simulink library "libc_filters_diff"  (R2013b)
settings: Solver=FixedStepDiscrete  StartTime=0.0  StopTime=Inf  FixedStep=0.004  RelTol=1e-3
PostLoadFcn:
  | , if any(exist('dsrtsu_mdlpostloadfcn', 'file') == [2, 3, 6]), try dsrtsu_mdlpostloadfcn('Execute', bdroot); catch fprintf('Error in PostLoadFcn (dsrtsu_mdlpostloadfcn) for model "%s":\n %s\n', bdroot, lasterr); end, end,
undefined symbols (not defined in the file or in its folder): accurate, CONST, dim, DiscIntNeverNeededParam, O
undefined symbols (not defined in the file): BHA
libraries: simulink x20, libc_filters_diff x8
settings Model: DSRTSU_INTERNAL_RTI_VER=440  DSRTSU_INTERNAL_RTI_TYPE=rti1005  DSRTSU_INTERNAL_RTIFPGA=30  Creator=Falkenhahn  LastModifiedBy=Falkenhahn

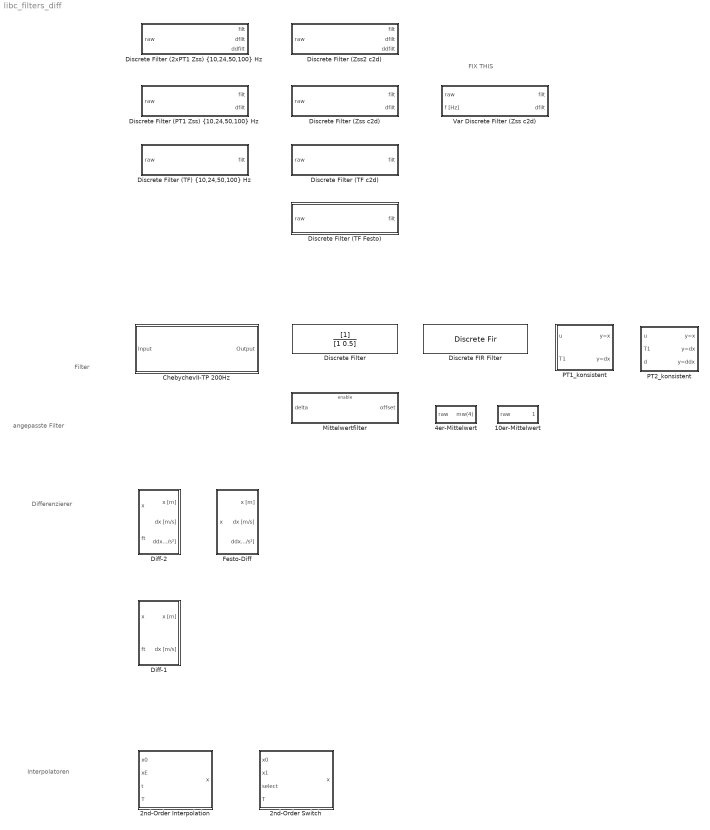
== system libc_filters_diff ==
  note: FIX THIS
  note: Filter
  note: Differenzierer
  note: angepasste Filter
  note: Interpolatoren
  10er-Mittelwert : Subsystem
      settings: AttributesFormatString=|
      | Mittelwert der
      | letzten 10 Werte
  2nd-Order Interpolation : Subsystem
  2nd-Order Switch : Subsystem
  4er-Mittelwert : Subsystem
      settings: AttributesFormatString=|
      | Mittelwert der
      | letzten 4 Werte
  ChebychevII-TP 200Hz : Subsystem  Tag=FilterWizardSubSystem  TreatAsAtomicUnit=on  SystemSampleTime=0.005
      settings: ErrorFcn=dspFilterRealizedInBasicElemsAlgLoopErrFcnCallback
      mask Display:
      | fprintf('Chebychev II-TP \n specified order: 4 \n F_Sample = 200 Hz \n F_Stopp = 25 Hz \n H_stopp^2<0.0001');
      | port_label('input', 1, 'vec-in');
      | port_label('output', 1, 'filt');
  Diff-1 : Subsystem  mask{fg=2.65}
      mask prompts: fg "Grenzfrequenz"
      mask help:
      | ft (feedthrough):
      | 0: phasengleichheit (maximal)
      | 1: phasenminimal
      settings: AttributesFormatString=f = %<fg>
  Diff-2 : Subsystem  mask{fg=2.65, D=1}
      mask prompts: fg "Grenzfrequenz fg"; D "Dämpfung D"
      mask help:
      | ft (feedthrough):
      | 0: phasengleichheit (maximal)
      | 1: phasenminimal
      |
      | D = 1 entspricht zwei PT1-Gliedern mit gleicher Zeitkonstante (kein Überschwingen)
      settings: AttributesFormatString=f = %<fg>\nD = %<D>
  Discrete FIR Filter : DiscreteFir
      settings: AttributesFormatString=sample time: %<SampleTime>
  Discrete Filter : DiscreteFilter
      settings: AttributesFormatString=sample time: %<SampleTime>
  "Discrete Filter (2xPT1 Zss) {10,24,50,100} Hz" : Subsystem  mask{rdnname2442_gf=10 Hz, rdnname2442_tA=CONST.tA}
      mask prompts: rdnname2442_gf "Grenzfrequenz"; rdnname2442_tA "Abstastzeit"
      mask init:
      | if rdnname2442_gf == 1 % first popup entry: 10 Hz
      |     rdnname2442_freq = 10;
      | elseif rdnname2442_gf == 2 % second popup entry: 24 Hz
      |     rdnname2442_freq = 24;
      | elseif rdnname2442_gf == 3 % third popup entry: 50 Hz
      |     rdnname2442_freq = 50;
      | else % rdnname2442_gf == 4 % third popup entry: 100 Hz
      |     rdnname2442_freq = 100;
      | end
      settings: AttributesFormatString=%<rdnname2442_gf>, tA: %<rdnname2442_tA>
      mask TypeOptions rdnname2442_gf: 10 Hz | 24 Hz | 50 Hz | 100 Hz
      mask Display: dpoly(1,[1/(2*pi*rdnname2442_freq) 1]);
  "Discrete Filter (PT1 Zss) {10,24,50,100} Hz" : Subsystem  mask{rdnname2442_gf=10 Hz, rdnname2442_tA=CONST.tA}
      mask prompts: rdnname2442_gf "Grenzfrequenz"; rdnname2442_tA "Abstastzeit"
      mask init: same as libc_filters_diff/Discrete Filter (2xPT1 Zss) {10,24,50,100} Hz
      settings: AttributesFormatString=%<rdnname2442_gf>, tA: %<rdnname2442_tA>
      mask TypeOptions rdnname2442_gf: 10 Hz | 24 Hz | 50 Hz | 100 Hz
      mask Display: dpoly(1,[1/(2*pi*rdnname2442_freq) 1])
  Discrete Filter (TF Festo) : Subsystem  mask{num_a=[1], den_a=[1/(2*pi*45), 1], Tsamp=CONST.tA, method='ramp', dar='z'}
      mask prompts: num_a "Numerator"; den_a "Denominator"; Tsamp "Abtastzeit, optional Abtastzeit für Diskret.  Ts  bzw.  [Ts,Ts_disk]"; method "Methode: Euler, Trapez, Heun, rK4, steP, step_U, Ramp, tr_100"; dar "Darstellung: z, z- = diskret, d = analoge ÜF des disk. Sys."
      mask init:
      | if length(Tsamp) == 0
      |     num_s = 0;
      |     num = 0;
      |     den_s = 1;
      |     den = 1;
      |     disp('ERROR: Abtastzeit nicht definiert. Ist CONST.tA definiert oder wurde die Abtastzeitvariable verändert?');
      | else
      |     Ts_int=Tsamp(1);
      |     if length(Tsamp)==1
      |         Ts=Tsamp(1); 
      |     else
      |         Ts=Tsamp(2);
      |     end
      |     if Ts == -1
      |         disp('ERROR: Abtastzeit für Diskretisierung = -1, Zweite Abtastzeit eingeben')
      |     end
      | 
      |     if exist('discret') == 2
      |         [a,b,c,d]=tf2ss(num_a,den_a); 
      |         [ad,bd,cd,dd,art]=discret(a,b,c,d,Ts,method,1e-9);
      |         [num,den]=ss2tf(ad,bd,cd,dd,1);
      |     else
      |         num_s = 0;
      |         num = 0;
      |         den_s = 1;
      |         den = 1;
      |         disp('ERROR: Festo tools initialisieren');
      |     end
      | 
      | 
      |     if dar(1) =='z'
      |         num_s=num; 
      |         den_s=den; 
      |     else
      |         num_s=num_a; 
      |         den_s=den_a; 
      |         if dar == 'd'
      |             dar = art
      |         end
      |     end
      | end
      settings: AttributesFormatString=sample time: %<Tsamp>
      mask Display:
      | if length(Tsamp) == 0
      |     disp('undefined sample time\n(e.g. CONST.tA)');
      | else
      |     if exist('discret') ~= 2
      |         disp('Festo tools not initialized');
      |     else
      |         dpoly(num_s,den_s,dar);
      |     end
      | end
  Discrete Filter (TF c2d) : Subsystem  mask(Diskretes Filter){rdnname2342_gf=45, rdnname2342_initial_cond=0, rdnname2342_tA=CONST.tA, rdnname2342_mode=noh (d=0), rdnname2342_showd=off}
      mask prompts: rdnname2342_gf "Grenzfrequenz [Hz]"; rdnname2342_initial_cond "Anfangsbedingungen"; rdnname2342_tA "Abtastzeit [s]"; rdnname2342_mode "Diskretisierung"; rdnname2342_showd "Diskrete Darstellung"
      mask init:
      | if rdnname2342_tA == 0
      |     error('invalid sample time');
      | end
      | if rdnname2342_gf == 0
      |     error('invalid cut-off frequency');
      | end
      | 
      | c_sys = tf(1,[1/(2*pi*rdnname2342_gf) 1]);
      | [rdnname2342_cnum,rdnname2342_cden] = tfdata(c_sys,'v');
      | 
      | rdnname2342_num = 1; % default value
      | rdnname2342_den = 1; % default value
      | if rdnname2342_mode == 3 % 'noh (d=0)'
      |     if exist('discret') == 2
      |         [a,b,c,d]=tf2ss(rdnname2342_cnum,rdnname2342_cden); 
      |         [ad,bd,cd,dd,art]=discret(a,b,c,d,rdnname2342_tA,'step_u',1e-9);
      |         [rdnname2342_num,rdnname2342_den]=ss2tf(ad,bd,cd,dd,1);
      |     else
      |         disp('ERROR: Festo tools initialisieren (fallback: foh (d=dt/2))'); 
      |         rdnname2342_mode = 2;
      |     end
      | end
      | if rdnname2342_mode == 2 % 'foh (d=dt/2)'
      |     d_sys = c2d(c_sys,rdnname2342_tA,'foh');
      |     [rdnname2342_num,rdnname2342_den] = tfdata(d_sys,'v');
      | end
      | if rdnname2342_mode == 1 % 'zoh (d=dt)'
      |     d_sys = c2d(c_sys,rdnname2342_tA);
      |     [rdnname2342_num,rdnname2342_den] = tfdata(d_sys,'v');
      | end
      settings: AttributesFormatString=%<rdnname2342_gf> Hz, IC: %<rdnname2342_initial_cond>, %<rdnname2342_mode>
      mask TypeOptions rdnname2342_mode: zoh (d=dt) | foh (d=dt/2) | noh (d=0)
      mask Display:
      | if rdnname2342_showd
      |     dpoly(rdnname2342_num,rdnname2342_den,'z')
      | else
      |     dpoly(rdnname2342_cnum,rdnname2342_cden);
      | end
  "Discrete Filter (TF) {10,24,50,100} Hz" : Subsystem  mask{rdnname2442_gf=10 Hz, rdnname2442_tA=CONST.tA, rdnname2442_IC=0}
      mask prompts: rdnname2442_gf "Grenzfrequenz"; rdnname2442_tA "Abstastzeit"; rdnname2442_IC "Anfangsbedingungen"
      mask init: same as libc_filters_diff/Discrete Filter (2xPT1 Zss) {10,24,50,100} Hz
      settings: AttributesFormatString=%<rdnname2442_gf>, IC: %<rdnname2442_IC>, tA: %<rdnname2442_tA>
      mask TypeOptions rdnname2442_gf: 10 Hz | 24 Hz | 50 Hz | 100 Hz
      mask Display: dpoly(1,[1/(2*pi*rdnname2442_freq) 1])
  Discrete Filter (Zss c2d) : Subsystem  mask(Diskretes Filter){rdnname2342_gf=45, rdnname2342_tA=CONST.tA, rdnname2342_mode=noh (d=0), rdnname2342_showd=on}
      mask prompts: rdnname2342_gf "Grenzfrequenz [Hz]"; rdnname2342_tA "Abtastzeit [s]"; rdnname2342_mode "Diskretisierung"; rdnname2342_showd "Diskrete Darstellung"
      mask init:
      | if rdnname2342_tA == 0
      |     error('invalid sample time');
      | end
      | if rdnname2342_gf == 0
      |     error('invalid cut-off frequency');
      | end
      | 
      | c_sys = tf(1,[1/(2*pi*rdnname2342_gf) 1]);
      | [rdnname2342_cnum,rdnname2342_cden] = tfdata(c_sys,'v');
      | 
      | rdnname2342_num = 1; % default value
      | rdnname2342_den = 1; % default value
      | if rdnname2342_mode == 3 % 'noh (d=0)'
      |     if exist('discret') == 2
      |         [a,b,c,d]=tf2ss(rdnname2342_cnum,rdnname2342_cden); 
      |         [ad,bd,cd,dd,art]=discret(a,b,c,d,rdnname2342_tA,'step_u',1e-9);
      |         [rdnname2342_num,rdnname2342_den]=ss2tf(ad,bd,cd,dd,1);
      |     else
      |         disp('ERROR: Festo tools initialisieren (fallback: foh (d=dt/2))'); 
      |         rdnname2342_mode = 2;
      |     end
      | end
      | if rdnname2342_mode == 2 % 'foh (d=dt/2)'
      |     d_sys = c2d(c_sys,rdnname2342_tA,'foh');
      |     [rdnname2342_num,rdnname2342_den] = tfdata(d_sys,'v');
      | end
      | if rdnname2342_mode == 1 % 'zoh (d=dt)'
      |     d_sys = c2d(c_sys,rdnname2342_tA);
      |     [rdnname2342_num,rdnname2342_den] = tfdata(d_sys,'v');
      | end
      | 
      | a = rdnname2342_den(2);
      | b = rdnname2342_den(1);
      | c = rdnname2342_num(2);
      | d = rdnname2342_num(1);
      settings: AttributesFormatString=%<rdnname2342_gf> Hz, %<rdnname2342_mode>
      mask TypeOptions rdnname2342_mode: zoh (d=dt) | foh (d=dt/2) | noh (d=0)
      mask Display:
      | if rdnname2342_showd
      |     dpoly(rdnname2342_num,rdnname2342_den,'z')
      | else
      |     dpoly(rdnname2342_cnum,rdnname2342_cden);
      | end
  Discrete Filter (Zss2 c2d) : Subsystem  mask(Diskretes Filter){rdnname2342_gf=45, rdnname2342_tA=CONST.tA, rdnname2342_mode=noh (d=0), rdnname2342_diffmode=O(2) [accurate], rdnname2342_showd=on}
      mask prompts: rdnname2342_gf "Grenzfrequenz [Hz]"; rdnname2342_tA "Abtastzeit [s]"; rdnname2342_mode "Diskretisierung"; rdnname2342_diffmode "Differenzierung"; rdnname2342_showd "Diskrete Darstellung"
      mask init: same as libc_filters_diff/Discrete Filter (Zss c2d)
      settings: AttributesFormatString=%<rdnname2342_gf> Hz, %<rdnname2342_mode>
      mask TypeOptions rdnname2342_mode: zoh (d=dt) | foh (d=dt/2) | noh (d=0)
      mask TypeOptions rdnname2342_diffmode: O(1) [low phase error] | O(2) [accurate]
      mask Display:
      | if rdnname2342_showd
      |     dpoly(rdnname2342_num,rdnname2342_den,'z');
      | else
      |     dpoly(rdnname2342_cnum,rdnname2342_cden);
      | end
  Festo-Diff : Subsystem
      settings: AttributesFormatString=mit PLC-Differenzierer
  Mittelwertfilter : Subsystem
      settings: AttributesFormatString=Eingangs-Mittelwertbildung wenn aktiviert,\nandernfalls wird Mittelwert gehalten & ausgegeben
  PT1_konsistent : Subsystem
  PT2_konsistent : Subsystem
  Var Discrete Filter (Zss c2d) : Subsystem  mask(Diskretes Filter){rdnname2342_tA=CONST.tA, rdnname2342_mode=noh (d=0)}
      mask prompts: rdnname2342_tA "Abtastzeit [s]"; rdnname2342_mode "Diskretisierung"
      mask init:
      | if rdnname2342_tA == 0
      |     error('invalid sample time');
      | end
      settings: AttributesFormatString=|
      | %<rdnname2342_mode>
      | CURRENTLY NOT USABLE FOR CODE GENERATION
      | BODE / C2D / TF ...
      mask TypeOptions rdnname2342_mode: zoh (d=dt) | foh (d=dt/2) | noh (d=0)
      mask Display: fprintf('!!!  FIX  ME !!!');

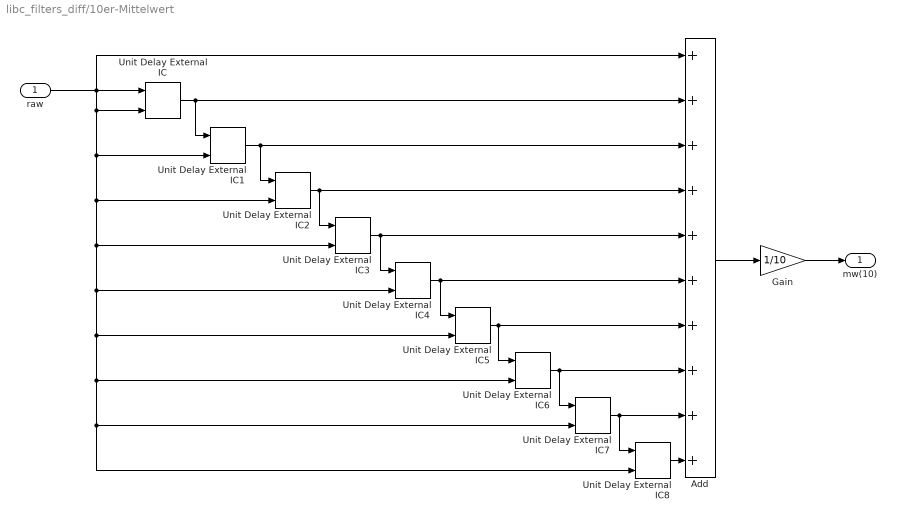
== system libc_filters_diff/10er-Mittelwert ==
  raw : Inport
  Add : Sum  Inputs=10
  Gain : Gain  Gain=1/10
  Unit Delay External IC{,1..8} (9 alike) : simulink/Additional Math & Discrete/Additional Discrete/Unit Delay External IC  tsamp=-1
  mw(10) : Outport  InitialOutput=zeros(1,dim)
  wires:
  Gain/1 -> mw(10)/1
  Add/1 -> Gain/1
  Unit Delay External IC2/1 -> Unit Delay External IC3/1, Add/4
  Unit Delay External IC1/1 -> Unit Delay External IC2/1, Add/3
  Unit Delay External IC/1 -> Add/2, Unit Delay External IC1/1
  raw/1 -> Unit Delay External IC/1, Add/1, Unit Delay External IC/2, Unit Delay External IC3/2, Unit Delay External IC4/2, Unit Delay External IC5/2, Unit Delay External IC6/2, Unit Delay External IC7/2, Unit Delay External IC8/2, Unit Delay External IC2/2, Unit Delay External IC1/2
  Unit Delay External IC8/1 -> Add/10
  Unit Delay External IC7/1 -> Add/9, Unit Delay External IC8/1
  Unit Delay External IC6/1 -> Add/8, Unit Delay External IC7/1
  Unit Delay External IC5/1 -> Unit Delay External IC6/1, Add/7
  Unit Delay External IC4/1 -> Unit Delay External IC5/1, Add/6
  Unit Delay External IC3/1 -> Add/5, Unit Delay External IC4/1

== system libc_filters_diff/2nd-Order Interpolation ==
  x0 : Inport
  xE : Inport  Port=2
  t : Inport  Port=3
  T : Inport  Port=4
  2nd-Order Interpolation : MATLAB Function  TreatAsAtomicUnit=on
  x : Outport
  wires:
  t/1 -> 2nd-Order Interpolation/3(t)
  2nd-Order Interpolation/1(x) -> x/1
  x0/1 -> 2nd-Order Interpolation/1(x0)
  xE/1 -> 2nd-Order Interpolation/2(xE)
  T/1 -> 2nd-Order Interpolation/4(T)

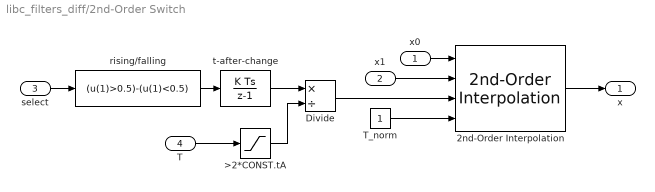
== system libc_filters_diff/2nd-Order Switch ==
  x0 : Inport
  x1 : Inport  Port=2
  select : Inport  Port=3
  T : Inport  Port=4
  2nd-Order Interpolation : libc_filters_diff/2nd-Order Interpolation
  >2*CONST.tA : Saturate  UpperLimit=inf  LowerLimit=2*CONST.tA
  Divide : Product  Inputs=*/
  T_norm : Constant
  rising/falling : Fcn  Expr=(u(1)>0.5)-(u(1)<0.5)
  t-after-change : DiscreteIntegrator  SampleTime=-1  LimitOutput=on  UpperSaturationLimit=1  LowerSaturationLimit=0  ICPrevOutput=DiscIntNeverNeededParam  ICPrevScaledInput=DiscIntNeverNeededParam
  x : Outport
  wires:
  2nd-Order Interpolation/1 -> x/1
  x0/1 -> 2nd-Order Interpolation/1
  x1/1 -> 2nd-Order Interpolation/2
  select/1 -> rising/falling/1
  Divide/1 -> 2nd-Order Interpolation/3
  rising/falling/1 -> t-after-change/1
  T_norm/1 -> 2nd-Order Interpolation/4
  >2*CONST.tA/1 -> Divide/2
  T/1 -> >2*CONST.tA/1
  t-after-change/1 -> Divide/1

== system libc_filters_diff/4er-Mittelwert ==
  raw : Inport
  Add : Sum  Inputs=++++
  Gain : Gain  Gain=1/4
  Unit Delay External IC : simulink/Additional Math & Discrete/Additional Discrete/Unit Delay External IC  tsamp=-1
  Unit Delay External IC1 : simulink/Additional Math & Discrete/Additional Discrete/Unit Delay External IC  tsamp=-1
  Unit Delay External IC2 : simulink/Additional Math & Discrete/Additional Discrete/Unit Delay External IC  tsamp=-1
  mw(4) : Outport  InitialOutput=zeros(1,dim)
  wires:
  raw/1 -> Unit Delay External IC1/2, Unit Delay External IC2/2, Unit Delay External IC/2, Add/1, Unit Delay External IC/1
  Unit Delay External IC/1 -> Unit Delay External IC1/1, Add/2
  Unit Delay External IC1/1 -> Add/3, Unit Delay External IC2/1
  Unit Delay External IC2/1 -> Add/4
  Add/1 -> Gain/1
  Gain/1 -> mw(4)/1

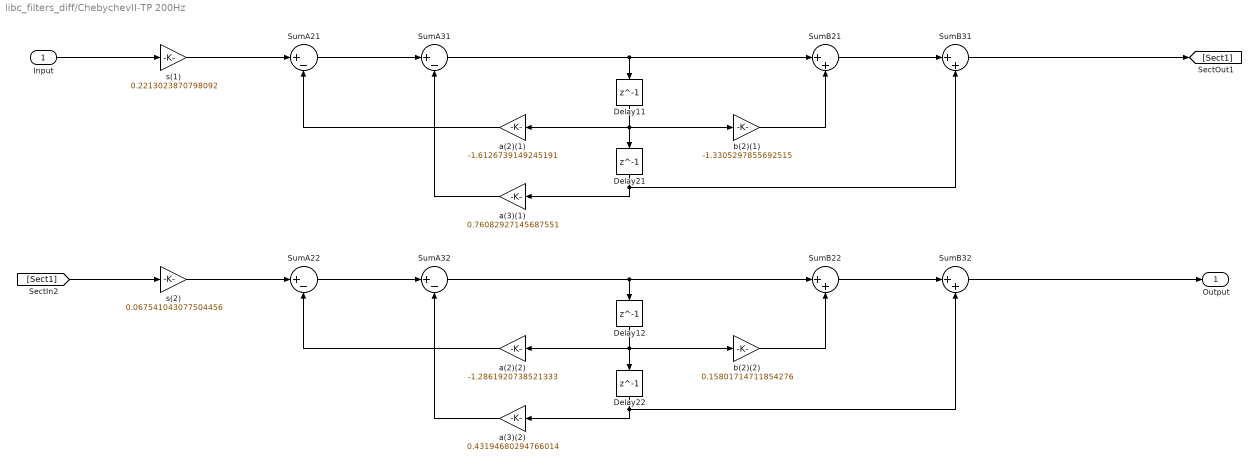
== system libc_filters_diff/ChebychevII-TP 200Hz ==
  Input : Inport
  Delay{11..12,21..22} (4 alike) : Delay  DelayLength=1  InitialCondition=0  InputProcessing=Inherited
  SumA{21..22,31..32} (4 alike) : Sum  Inputs=|+-  RndMeth=Nearest  SaturateOnIntegerOverflow=on  OutDataTypeStr=Inherit: Same as first input
  SumB{21..22,31..32} (4 alike) : Sum  Inputs=|++  RndMeth=Nearest  SaturateOnIntegerOverflow=on  OutDataTypeStr=Inherit: Same as first input
  a(2)(1) : Gain  Gain=-1.6126739149245191  ParamDataTypeStr=float('double')  RndMeth=Nearest  SaturateOnIntegerOverflow=on  OutDataTypeStr=Inherit: Same as input
  a(2)(2) : Gain  Gain=-1.2861920738521333  ParamDataTypeStr=float('double')  RndMeth=Nearest  SaturateOnIntegerOverflow=on  OutDataTypeStr=Inherit: Same as input
  a(3)(1) : Gain  Gain=0.76082927145687551  ParamDataTypeStr=float('double')  RndMeth=Nearest  SaturateOnIntegerOverflow=on  OutDataTypeStr=Inherit: Same as input
  a(3)(2) : Gain  Gain=0.43194680294766014  ParamDataTypeStr=float('double')  RndMeth=Nearest  SaturateOnIntegerOverflow=on  OutDataTypeStr=Inherit: Same as input
  b(2)(1) : Gain  Gain=-1.3305297855692515  ParamDataTypeStr=float('double')  RndMeth=Nearest  SaturateOnIntegerOverflow=on  OutDataTypeStr=Inherit: Same as input
  b(2)(2) : Gain  Gain=0.15801714711854276  ParamDataTypeStr=float('double')  RndMeth=Nearest  SaturateOnIntegerOverflow=on  OutDataTypeStr=Inherit: Same as input
  s(1) : Gain  Gain=0.2213023870798092  ParamDataTypeStr=float('double')  RndMeth=Nearest  SaturateOnIntegerOverflow=on  OutDataTypeStr=Inherit: Same as input
  s(2) : Gain  Gain=0.067541043077504456  ParamDataTypeStr=float('double')  RndMeth=Nearest  SaturateOnIntegerOverflow=on  OutDataTypeStr=Inherit: Same as input
  Output : Outport
  wires:
  Delay22/1 -> SumB32/2, a(3)(2)/1
  a(3)(2)/1 -> SumA32/2
  b(2)(2)/1 -> SumB22/2
  Delay12/1 -> Delay22/1, b(2)(2)/1, a(2)(2)/1
  a(2)(2)/1 -> SumA22/2
  SumB32/1 -> Output/1
  SumB22/1 -> SumB32/1
  SumA32/1 -> Delay12/1, SumB22/1
  SumA22/1 -> SumA32/1
  s(2)/1 -> SumA22/1
  [Sect1] -> s(2)/1
  Delay21/1 -> SumB31/2, a(3)(1)/1
  a(3)(1)/1 -> SumA31/2
  b(2)(1)/1 -> SumB21/2
  Delay11/1 -> Delay21/1, b(2)(1)/1, a(2)(1)/1
  a(2)(1)/1 -> SumA21/2
  SumB31/1 -> [Sect1]
  SumB21/1 -> SumB31/1
  SumA31/1 -> Delay11/1, SumB21/1
  SumA21/1 -> SumA31/1
  s(1)/1 -> SumA21/1
  Input/1 -> s(1)/1

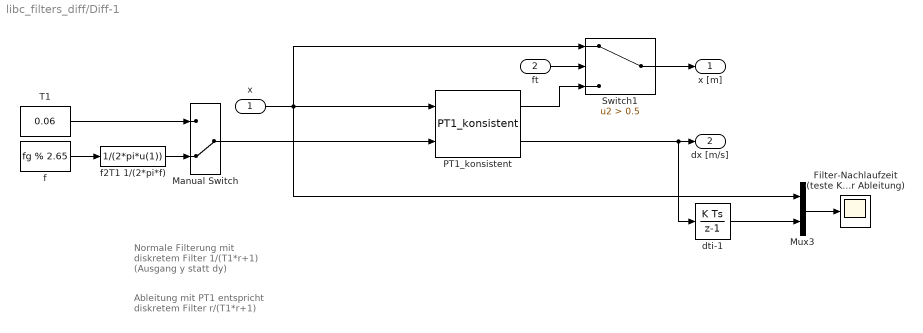
== system libc_filters_diff/Diff-1 ==
  note: Normale Filterung mit
      | diskretem Filter 1/(T1*r+1)
      | (Ausgang y statt dy)
  note: Ableitung mit PT1 entspricht
      | diskretem Filter r/(T1*r+1)
  x : Inport
  ft : Inport  Port=2
  Filter-Nachlaufzeit (teste Konsistenz der Ableitung) : Scope
      settings: TimeRange=10  YMin=0.22  YMax=0.2625  SaveName=ScopeData6
  Manual Switch : ManualSwitch  CurrentSetting=0
  Mux3 : Mux  Inputs=2
  PT1_konsistent : libc_filters_diff/PT1_konsistent
  Switch1 : Switch  Criteria=u2 > Threshold  Threshold=0.5
  T1 : Constant  Value=0.06
  dti-1 : DiscreteIntegrator  SampleTime=-1  ICPrevOutput=DiscIntNeverNeededParam  ICPrevScaledInput=DiscIntNeverNeededParam
  f : Constant  Value=fg % 2.65
  f2T1 1/(2*pi*f) : Fcn  Expr=1/(2*pi*u(1))
  x [m] : Outport
  dx [m/s] : Outport  Port=2
  wires:
  PT1_konsistent/2 -> dti-1/1, dx [m/s]/1
  Switch1/1 -> x [m]/1
  ft/1 -> Switch1/2
  f/1 -> f2T1 1/(2*pi*f)/1
  f2T1 1/(2*pi*f)/1 -> Manual Switch/2
  T1/1 -> Manual Switch/1
  x/1 -> Mux3/1, Switch1/1, PT1_konsistent/1
  dti-1/1 -> Mux3/2
  Mux3/1 -> Filter-Nachlaufzeit (teste Konsistenz der Ableitung)/1
  PT1_konsistent/1 -> Switch1/3
  Manual Switch/1 -> PT1_konsistent/2

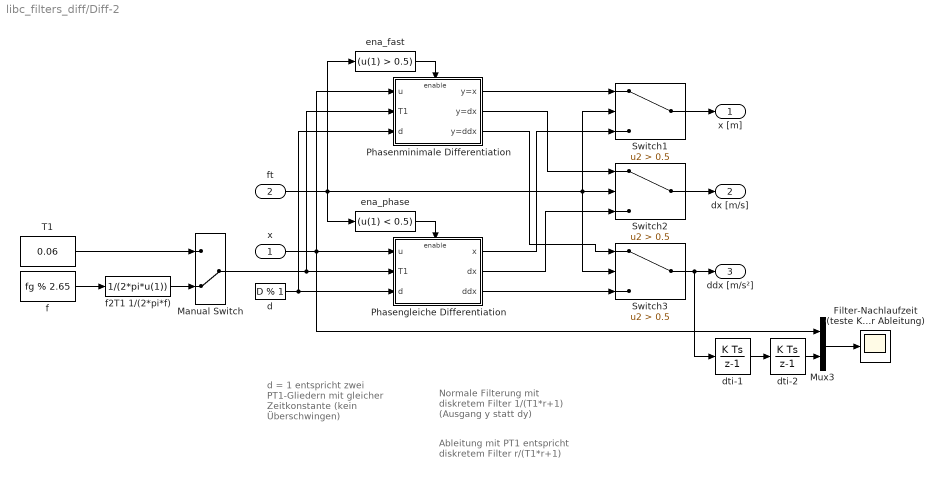
== system libc_filters_diff/Diff-2 ==
  note: Ableitung mit PT1 entspricht
      | diskretem Filter r/(T1*r+1)
  note: Normale Filterung mit
      | diskretem Filter 1/(T1*r+1)
      | (Ausgang y statt dy)
  note: d = 1
      | entspricht zwei PT1-Gliedern mit
      | gleicher Zeitkonstante
      | (kein Überschwingen)
  x : Inport
  ft : Inport  Port=2
  Filter-Nachlaufzeit (teste Konsistenz der Ableitung) : Scope
      settings: TimeRange=10  YMin=0.22  YMax=0.2625  SaveName=ScopeData6
  Manual Switch : ManualSwitch  CurrentSetting=0
  Mux3 : Mux  Inputs=2
  Phasengleiche Differentiation : Subsystem
  Phasenminimale Differentiation : Subsystem
  Switch1 : Switch  Criteria=u2 > Threshold  Threshold=0.5
  Switch2 : Switch  Criteria=u2 > Threshold  Threshold=0.5
  Switch3 : Switch  Criteria=u2 > Threshold  Threshold=0.5
  T1 : Constant  Value=0.06
  d : Constant  Value=D % 1
  dti-1 : DiscreteIntegrator  SampleTime=-1  ICPrevOutput=DiscIntNeverNeededParam  ICPrevScaledInput=DiscIntNeverNeededParam
  dti-2 : DiscreteIntegrator  SampleTime=-1  ICPrevOutput=DiscIntNeverNeededParam  ICPrevScaledInput=DiscIntNeverNeededParam
  ena_fast : Fcn  Expr=(u(1) > 0.5)
  ena_phase : Fcn  Expr=(u(1) < 0.5)
  f : Constant  Value=fg % 2.65
  f2T1 1/(2*pi*f) : Fcn  Expr=1/(2*pi*u(1))
  x [m] : Outport
  dx [m/s] : Outport  Port=2
  ddx [m/s²] : Outport  Port=3
  wires:
  Mux3/1 -> Filter-Nachlaufzeit (teste Konsistenz der Ableitung)/1
  dti-2/1 -> Mux3/2
  dti-1/1 -> dti-2/1
  x/1 -> Mux3/1, Phasenminimale Differentiation/1(u), Phasengleiche Differentiation/1(u)
  T1/1 -> Manual Switch/1
  f2T1 1/(2*pi*f)/1 -> Manual Switch/2
  f/1 -> f2T1 1/(2*pi*f)/1
  Manual Switch/1 -> Phasenminimale Differentiation/2(T1), Phasengleiche Differentiation/2(T1)
  d/1 -> Phasenminimale Differentiation/3(d), Phasengleiche Differentiation/3(d)
  Phasenminimale Differentiation/1(y=x) -> Switch1/1
  Phasengleiche Differentiation/1(x) -> Switch1/3
  Phasengleiche Differentiation/3(ddx) -> Switch3/3
  Phasengleiche Differentiation/2(dx) -> Switch2/3
  Phasenminimale Differentiation/2(y=dx) -> Switch2/1
  Phasenminimale Differentiation/3(y=ddx) -> Switch3/1
  ena_fast/1 -> Phasenminimale Differentiation/Enable
  ena_phase/1 -> Phasengleiche Differentiation/Enable
  ft/1 -> ena_fast/1, Switch3/2, Switch1/2, Switch2/2, ena_phase/1
  Switch1/1 -> x [m]/1
  Switch2/1 -> dx [m/s]/1
  Switch3/1 -> dti-1/1, ddx [m/s²]/1

== system libc_filters_diff/Discrete Filter (2xPT1 Zss) {10,24,50,100} Hz ==
  note: zum Filtern am besten geeignet
      | (da kein Phasenverlust): noh (d=0)
  raw : Inport
  Discrete Filter (Zss2 c2d) : libc_filters_diff/Discrete Filter (Zss2 c2d)  rdnname2342_gf=rdnname2442_freq  rdnname2342_tA=rdnname2442_tA  rdnname2342_mode=noh (d=0)  rdnname2342_diffmode=O(2) [accurate]  rdnname2342_showd=on
      settings: AttributesFormatString=%<rdnname2342_gf> Hz, %<rdnname2342_mode>
  filt : Outport
  dfilt : Outport  Port=2
  ddfilt : Outport  Port=3
  wires:
  Discrete Filter (Zss2 c2d)/2 -> dfilt/1
  raw/1 -> Discrete Filter (Zss2 c2d)/1
  Discrete Filter (Zss2 c2d)/1 -> filt/1
  Discrete Filter (Zss2 c2d)/3 -> ddfilt/1

== system libc_filters_diff/Discrete Filter (PT1 Zss) {10,24,50,100} Hz ==
  note: zum Filtern am besten geeignet
      | (da kein Phasenverlust): noh (d=0)
  raw : Inport
  Discrete Filter (Zss c2d) : libc_filters_diff/Discrete Filter (Zss c2d)  rdnname2342_gf=rdnname2442_freq  rdnname2342_tA=rdnname2442_tA  rdnname2342_mode=noh (d=0)  rdnname2342_showd=on
      settings: AttributesFormatString=%<rdnname2342_gf> Hz, %<rdnname2342_mode>
  filt : Outport
  dfilt : Outport  Port=2
  wires:
  Discrete Filter (Zss c2d)/1 -> filt/1
  raw/1 -> Discrete Filter (Zss c2d)/1
  Discrete Filter (Zss c2d)/2 -> dfilt/1

== system libc_filters_diff/Discrete Filter (TF Festo) ==
  raw : Inport
  Discrete Transfer Fcn : DiscreteTransferFcn  Numerator=num  Denominator=den  SampleTime=Ts_int
  filt : Outport
  wires:
  raw/1 -> Discrete Transfer Fcn/1
  Discrete Transfer Fcn/1 -> filt/1

== system libc_filters_diff/Discrete Filter (TF c2d) ==
  raw : Inport
  Diskretes Filter : DiscreteTransferFcn  Numerator=rdnname2342_num  Denominator=rdnname2342_den  InitialStates=rdnname2342_initial_cond  ExternalReset=Rising  SampleTime=rdnname2342_tA
      settings: InputPortMap=u0,r7
  reset : Constant  Value=0
  filt : Outport
  wires:
  reset/1 -> Diskretes Filter/2
  raw/1 -> Diskretes Filter/1
  Diskretes Filter/1 -> filt/1

== system libc_filters_diff/Discrete Filter (TF) {10,24,50,100} Hz ==
  note: zum Filtern am besten geeignet
      | (da kein Phasenverlust): noh (d=0)
  raw : Inport
  Discrete Filter (TF c2d) : libc_filters_diff/Discrete Filter (TF c2d)  rdnname2342_gf=rdnname2442_freq  rdnname2342_initial_cond=rdnname2442_IC  rdnname2342_tA=rdnname2442_tA  rdnname2342_mode=noh (d=0)  rdnname2342_showd=on
      settings: AttributesFormatString=%<rdnname2342_gf> Hz, IC: %<rdnname2342_initial_cond>, %<rdnname2342_mode>
  filt : Outport
  wires:
  raw/1 -> Discrete Filter (TF c2d)/1
  Discrete Filter (TF c2d)/1 -> filt/1

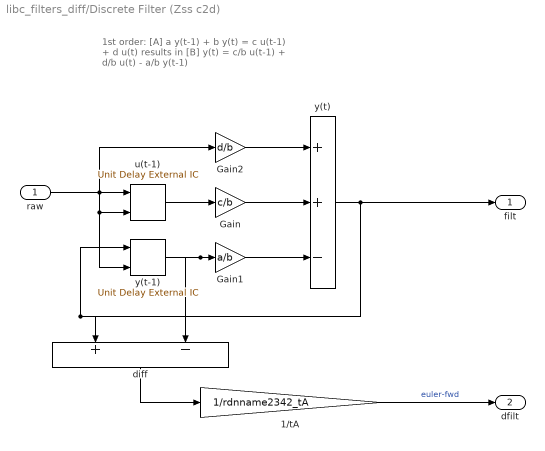
== system libc_filters_diff/Discrete Filter (Zss c2d) ==
  note: 1st order:
      | [A]  a y(t-1) + b y(t) = c u(t-1) + d u(t)
      | results in
      | [B]  y(t) = c/b u(t-1) + d/b u(t) - a/b y(t-1)
  raw : Inport
  1/tA : Gain  Gain=1/rdnname2342_tA
  Gain : Gain  Gain=c/b
  Gain1 : Gain  Gain=a/b
  Gain2 : Gain  Gain=d/b
  diff : Sum  Inputs=+|-
  u(t-1) : simulink/Additional Math & Discrete/Additional Discrete/Unit Delay External IC  tsamp=rdnname2342_tA
  y(t) : Sum  Inputs=++-
  y(t-1) : simulink/Additional Math & Discrete/Additional Discrete/Unit Delay External IC  tsamp=rdnname2342_tA
  filt : Outport
  dfilt : Outport  Port=2
  wires:
  1/tA/1 -> dfilt/1  "euler-fwd"
  diff/1 -> 1/tA/1
  raw/1 -> u(t-1)/1, u(t-1)/2, y(t-1)/2, Gain2/1
  y(t)/1 -> diff/1, y(t-1)/1, filt/1
  Gain1/1 -> y(t)/3
  Gain/1 -> y(t)/2
  Gain2/1 -> y(t)/1
  y(t-1)/1 -> diff/2, Gain1/1
  u(t-1)/1 -> Gain/1

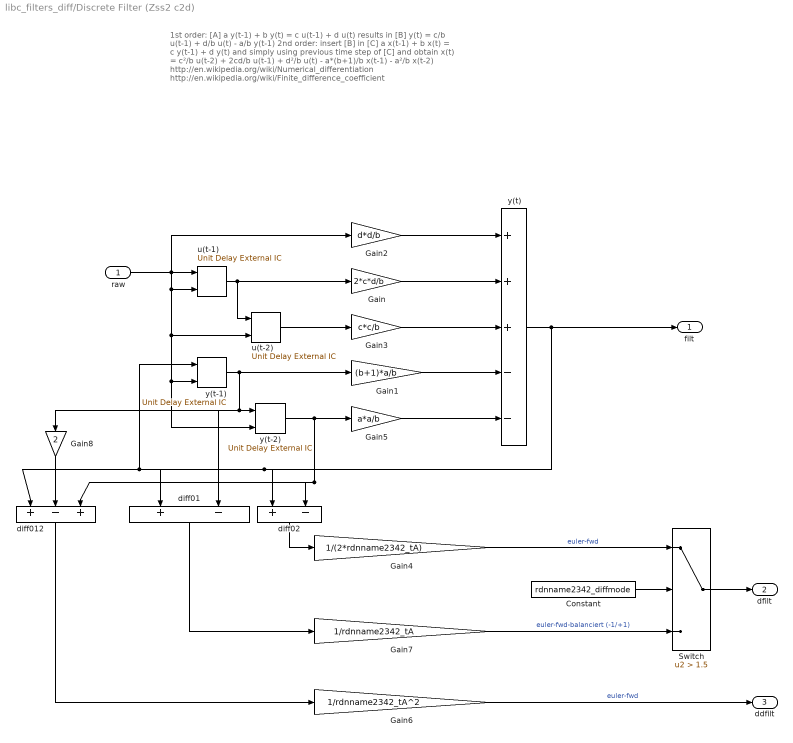
== system libc_filters_diff/Discrete Filter (Zss2 c2d) ==
  note: 1st order:
      | [A]  a y(t-1) + b y(t) = c u(t-1) + d u(t)
      | results in
      | [B]  y(t) = c/b u(t-1) + d/b u(t) - a/b y(t-1)
      |
      | 2nd order:  insert [B] in
      | [C]  a x(t-1) + b x(t) = c y(t-1) + d y(t)
      | and simply using previous time step of [C] and obtain
      | x(t) = c²/b u(t-2) + 2cd/b u(t-1) + d²/b u(t) - a*(b+1)/b x(t-1) - a²/b x(t-2)
      |
      | http://en.wikipedia.org/wiki/Numerical_differentiation
      | http://en.wikipedia.org/wiki/Finite_difference_coefficient
  raw : Inport
  Constant : Constant  Value=rdnname2342_diffmode
  Gain : Gain  Gain=2*c*d/b
  Gain1 : Gain  Gain=(b+1)*a/b
  Gain2 : Gain  Gain=d*d/b
  Gain3 : Gain  Gain=c*c/b
  Gain4 : Gain  Gain=1/(2*rdnname2342_tA)
  Gain5 : Gain  Gain=a*a/b
  Gain6 : Gain  Gain=1/rdnname2342_tA^2
  Gain7 : Gain  Gain=1/rdnname2342_tA
  Gain8 : Gain  Gain=2
  Switch : Switch  Criteria=u2 > Threshold  Threshold=1.5
  diff01 : Sum  Inputs=+|||-
  diff012 : Sum  Inputs=+|-|+
  diff02 : Sum  Inputs=+|||-
  u(t-1) : simulink/Additional Math & Discrete/Additional Discrete/Unit Delay External IC  tsamp=rdnname2342_tA
  u(t-2) : simulink/Additional Math & Discrete/Additional Discrete/Unit Delay External IC  tsamp=rdnname2342_tA
  y(t) : Sum  Inputs=+++--
  y(t-1) : simulink/Additional Math & Discrete/Additional Discrete/Unit Delay External IC  tsamp=rdnname2342_tA
  y(t-2) : simulink/Additional Math & Discrete/Additional Discrete/Unit Delay External IC  tsamp=rdnname2342_tA
  filt : Outport
  dfilt : Outport  Port=2
  ddfilt : Outport  Port=3
  wires:
  u(t-1)/1 -> u(t-2)/1, Gain/1
  y(t-1)/1 -> Gain1/1, Gain8/1, diff01/2, y(t-2)/1
  y(t)/1 -> y(t-1)/1, diff01/1, diff012/1, diff02/1, filt/1
  raw/1 -> Gain2/1, y(t-1)/2, y(t-2)/2, u(t-2)/2, u(t-1)/2, u(t-1)/1
  diff02/1 -> Gain4/1
  Gain4/1 -> Switch/1  "euler-fwd"
  u(t-2)/1 -> Gain3/1
  y(t-2)/1 -> Gain5/1, diff012/3, diff02/2
  Gain1/1 -> y(t)/4
  Gain3/1 -> y(t)/3
  Gain/1 -> y(t)/2
  Gain2/1 -> y(t)/1
  Gain5/1 -> y(t)/5
  Gain6/1 -> ddfilt/1  "euler-fwd"
  diff01/1 -> Gain7/1
  Gain7/1 -> Switch/3  "euler-fwd-balanciert (-1/+1)"
  Switch/1 -> dfilt/1
  Gain8/1 -> diff012/2
  diff012/1 -> Gain6/1
  Constant/1 -> Switch/2

== system libc_filters_diff/Festo-Diff ==
  x : Inport
  For Each Subsystem : Subsystem  TreatAsAtomicUnit=on
  Permute Dimensions : PermuteDimensions
  Permute Dimensions1 : PermuteDimensions
  Selector : Selector  NumberOfDimensions=2  InputPortWidth=3  IndexOptions=Index vector (dialog),Select all  Indices=[1],1  OutputSizes=1,1
  Selector1 : Selector  NumberOfDimensions=2  InputPortWidth=3  IndexOptions=Index vector (dialog),Select all  Indices=[2],1  OutputSizes=1,1
  x [m] : Outport
  dx [m/s] : Outport  Port=2
  ddx [m/s²] : Outport  Port=3
  wires:
  Permute Dimensions1/1 -> dx [m/s]/1
  Permute Dimensions/1 -> ddx [m/s²]/1
  Selector1/1 -> Permute Dimensions/1
  For Each Subsystem/1("[x dx ddx]") -> Selector/1, Selector1/1
  x/1 -> For Each Subsystem/1(x), x [m]/1
  Selector/1 -> Permute Dimensions1/1

== system libc_filters_diff/Mittelwertfilter ==
  delta : Inport
  Enable : EnablePort  StatesWhenEnabling=reset
  Add1 : Sum  Inputs=+++
  Add2 : Sum
  Constant : Constant
  Divide : Product  Inputs=*/
  Unit Delay : UnitDelay  SampleTime=-1
  Unit Delay2 : UnitDelay  SampleTime=-1
  size : Gain  Gain=0
  offset : Outport  InitialOutput=0
  wires:
  size/1 -> Add1/1
  Constant/1 -> Add1/2
  Add1/1 -> Divide/2, Unit Delay2/1
  Unit Delay2/1 -> Add1/3
  Add2/1 -> Unit Delay/1, Divide/1
  Unit Delay/1 -> Add2/2
  delta/1 -> Add2/1, size/1
  Divide/1 -> offset/1

== system libc_filters_diff/PT1_konsistent ==
  u : Inport
  T1 : Inport  Port=2
  Add2 : Sum  Inputs=+-
  Product : Product  Inputs=*/  RndMeth=Zero
  dti2 : DiscreteIntegrator  InitialConditionSource=external  SampleTime=-1  ICPrevOutput=DiscIntNeverNeededParam  ICPrevScaledInput=DiscIntNeverNeededParam
  y=x : Outport
  y=dx : Outport  Port=2
  wires:
  u/1 -> Add2/1, dti2/2
  dti2/1 -> y=x/1, Add2/2
  Add2/1 -> Product/1
  T1/1 -> Product/2
  Product/1 -> dti2/1, y=dx/1

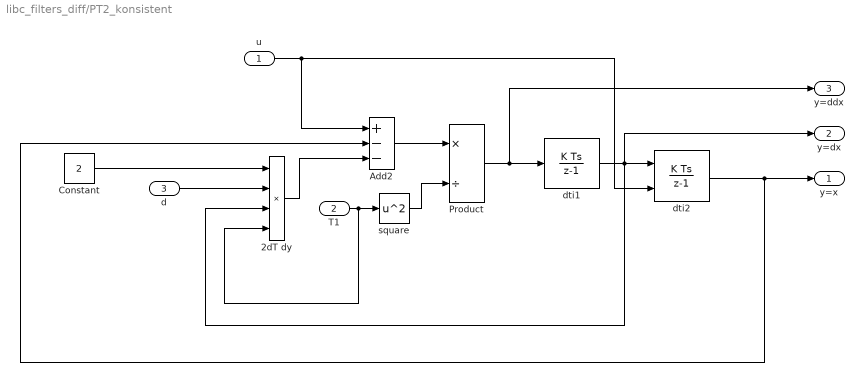
== system libc_filters_diff/PT2_konsistent ==
  u : Inport
  T1 : Inport  Port=2
  d : Inport  Port=3
  2dT dy : Product  Inputs=****  RndMeth=Zero
  Add2 : Sum  Inputs=+--
  Constant : Constant  Value=2
  Product : Product  Inputs=*/  RndMeth=Zero
  dti1 : DiscreteIntegrator  SampleTime=-1  ICPrevOutput=DiscIntNeverNeededParam  ICPrevScaledInput=DiscIntNeverNeededParam
  dti2 : DiscreteIntegrator  InitialConditionSource=external  InitialCondition=0.174  SampleTime=-1  ICPrevOutput=DiscIntNeverNeededParam  ICPrevScaledInput=DiscIntNeverNeededParam
  square : Math  Operator=square  SaturateOnIntegerOverflow=on
  y=x : Outport
  y=dx : Outport  Port=2
  y=ddx : Outport  Port=3
  wires:
  d/1 -> 2dT dy/2
  Constant/1 -> 2dT dy/1
  2dT dy/1 -> Add2/3
  square/1 -> Product/2
  dti1/1 -> dti2/1, y=dx/1, 2dT dy/3
  T1/1 -> 2dT dy/4, square/1
  Add2/1 -> Product/1
  Product/1 -> dti1/1, y=ddx/1
  dti2/1 -> Add2/2, y=x/1
  u/1 -> dti2/2, Add2/1

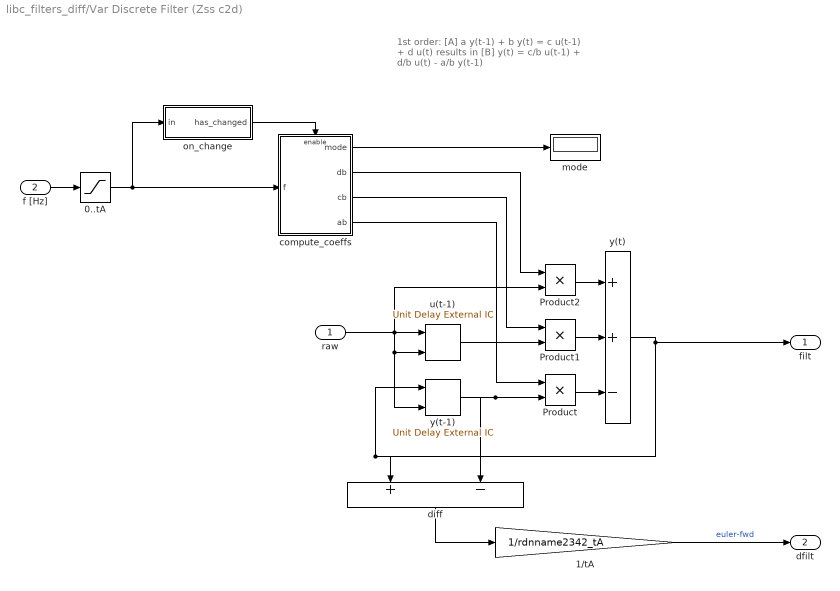
== system libc_filters_diff/Var Discrete Filter (Zss c2d) ==
  note: 1st order:
      | [A]  a y(t-1) + b y(t) = c u(t-1) + d u(t)
      | results in
      | [B]  y(t) = c/b u(t-1) + d/b u(t) - a/b y(t-1)
  raw : Inport
  f [Hz] : Inport  Port=2
  0..tA : Saturate  UpperLimit=1/rdnname2342_tA  LowerLimit=0.00000001
  1/tA : Gain  Gain=1/rdnname2342_tA
  Product : Product
  Product1 : Product
  Product2 : Product
  compute_coeffs : Subsystem
  diff : Sum  Inputs=+|-
  mode : Display
  on_change : Subsystem
  u(t-1) : simulink/Additional Math & Discrete/Additional Discrete/Unit Delay External IC  tsamp=rdnname2342_tA
  y(t) : Sum  Inputs=++-
  y(t-1) : simulink/Additional Math & Discrete/Additional Discrete/Unit Delay External IC  tsamp=rdnname2342_tA
  filt : Outport
  dfilt : Outport  Port=2
  wires:
  u(t-1)/1 -> Product1/2
  y(t-1)/1 -> Product/2, diff/2
  Product2/1 -> y(t)/1
  Product1/1 -> y(t)/2
  Product/1 -> y(t)/3
  y(t)/1 -> filt/1, y(t-1)/1, diff/1
  raw/1 -> Product2/2, y(t-1)/2, u(t-1)/2, u(t-1)/1
  diff/1 -> 1/tA/1
  1/tA/1 -> dfilt/1  "euler-fwd"
  f [Hz]/1 -> 0..tA/1
  0..tA/1 -> on_change/1(in), compute_coeffs/1(f)
  on_change/1(has_changed) -> compute_coeffs/Enable
  compute_coeffs/4(ab) -> Product/1
  compute_coeffs/3(cb) -> Product1/1
  compute_coeffs/2(db) -> Product2/1
  compute_coeffs/1(mode) -> mode/1

== system libc_filters_diff/Diff-2/Phasengleiche Differentiation ==
  note: Phasenkonsistente Ableitung.
      | Signale werden mit konsistenter
      | Filterzeit bearbeitet und
      | (untereinander) phasengleich
      | ausgegeben
  u : Inport
  T1 : Inport  Port=2
  d : Inport  Port=3
  Enable : EnablePort  PropagateVarSize=During execution
  PT2_konsistent : libc_filters_diff/PT2_konsistent
  x : Outport  InitialOutput=0.174
  dx : Outport  Port=2  InitialOutput=0
  ddx : Outport  Port=3  InitialOutput=0
  wires:
  PT2_konsistent/1 -> x/1
  PT2_konsistent/2 -> dx/1
  T1/1 -> PT2_konsistent/2
  d/1 -> PT2_konsistent/3
  u/1 -> PT2_konsistent/1
  PT2_konsistent/3 -> ddx/1

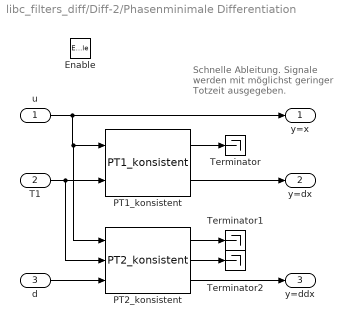
== system libc_filters_diff/Diff-2/Phasenminimale Differentiation ==
  note: Schnelle Ableitung.
      | Signale werden mit
      | möglichst geringer
      | Totzeit ausgegeben.
  u : Inport
  T1 : Inport  Port=2
  d : Inport  Port=3
  Enable : EnablePort  PropagateVarSize=During execution
  PT1_konsistent : libc_filters_diff/PT1_konsistent
  PT2_konsistent : libc_filters_diff/PT2_konsistent
  Terminator : Terminator
  Terminator1 : Terminator
  Terminator2 : Terminator
  y=x : Outport  InitialOutput=0.174
  y=dx : Outport  Port=2  InitialOutput=0
  y=ddx : Outport  Port=3  InitialOutput=0
  wires:
  u/1 -> PT1_konsistent/1, PT2_konsistent/1, y=x/1
  T1/1 -> PT1_konsistent/2, PT2_konsistent/2
  PT1_konsistent/1 -> Terminator/1
  PT1_konsistent/2 -> y=dx/1
  d/1 -> PT2_konsistent/3
  PT2_konsistent/3 -> y=ddx/1
  PT2_konsistent/2 -> Terminator2/1
  PT2_konsistent/1 -> Terminator1/1

== system libc_filters_diff/Festo-Diff/For Each Subsystem ==
  x : Inport  Partition=on  PartitionDimension=1  PartitionWidth=1
  For Each : ForEach  DisableCoverage=on  IndexMode=One-based
  PLC Differenzierer1 : Subsystem  mask{tA=CONST.tA, n=2, tv=0.005, x_ini=sum(BHA.Kin.l_ik_init)/3}
      mask prompts: tA "Abtastzeit"; n "Filterfaktor"; tv "Zeitkonstante Geschwindigkeitsausgang"; x_ini "Initialisierungsposition"
      mask help: Diskreter Differenzierer
      mask init:
      | str1=['Ts = ',n2s(tA*1000),' ms'];  str2=['n_filt = ',n2s(n)]; str3=['F_bw = ',n2s(1/(2.5*n*tA)),' Hz'];
      | abk=(4*n^2+2*n+1);
      | abk1=(2*n+1);
      | n2=n^2;
      | tA2=tA^2;
      | tv2=2*tv+tA;
      |  a11 = (2*n-1)/abk1;
      |   a12 = 0;
      |   a13 = 0;
      |   a21 = 4*n/abk1/abk;
      |   a22 = (4*n2+2*n-1)/abk;
      |   a23 = 4*n2*tA/abk;
      |   a31 = 8/tA*n/abk1/abk;
      |   a32 = -4/abk/tA;
      |   a33 = (4*n2-2*n-1)/abk;
      |   a44 = -(-2*tv+tA)/tv2;
      |   b11 = (2*n-1)/abk1^2+1/abk1;
      |   b21 = (40*n*n2+24*n2+4*n-1)/abk1^2/abk^2+1/abk1/abk;
      |   b31 = 2*(24*n*n2+8*n2-4*n-3)/tA/abk1^2/abk^2+2/abk1/abk/tA;
      |   b41 = 4*tA*tv/tv2^2;
      |   c11 =  -1/tA/n;     % old  c11 = 0;
      |   c12 = 0;
      |   c13 = 0;                % old  c13 = 1;
      |   c21 = 1/tA2/n2;
      |   c22 = -1/tA2/n2;
      |   c23 = -1/tA/n;
      |   c34 = -1/tv;
      |   d11 =  -1/tA/n/abk1+1/tA/n;     % old  d11 = 2/abk1/abk/tA;
      |   d21 = 4/tA2/abk1/abk;
      |   d31 = 2/tv2;
      | 
      | x1i =  2.0*n/abk1*x_ini;
      |  x2i =  4.0*n*(2.0*n*n+2.0*n+1.0)/abk1/abk*x_ini;
      |  x3i = -2.0/abk1/abk/tA*x_ini;
      |  x4i =  2.0*tv/tv2*x_ini;
      | 
      |  A_diff = [a11,a12,a13,0; a21,a22,a23,0; a31,a32,a33,0; 0,0,0,a44];
      | B_diff = [b11; b21; b31; b41];
      | C_diff = [c11,c12,c13,0; c21,c22,c23,0; 0,0,0,c34];
      | D_diff = [d11; d21; d31];
      | x0_diff = [x1i, x2i, x3i, x4i];
      mask Display: disp([str1,'\n',str2,'\n',str3])
  "[x dx ddx]" : Outport  ConcatenationDimension=2
  wires:
  PLC Differenzierer1/1("[v a]_diff") -> "[x dx ddx]"/1
  x/1 -> PLC Differenzierer1/1(x)

== system libc_filters_diff/Var Discrete Filter (Zss c2d)/compute_coeffs ==
  f : Inport
  Enable : EnablePort
  Constant : Constant  Value=rdnname2342_tA
  Constant1 : Constant  Value=rdnname2342_mode
  compute_coeffs : MATLAB Function  TreatAsAtomicUnit=on
  mode : Outport
  db : Outport  Port=2
  cb : Outport  Port=3
  ab : Outport  Port=4
  wires:
  f/1 -> compute_coeffs/1(f)
  compute_coeffs/4(ab) -> ab/1
  compute_coeffs/2(db) -> db/1
  compute_coeffs/3(cb) -> cb/1
  compute_coeffs/1(cmode) -> mode/1
  Constant/1 -> compute_coeffs/2(tA)
  Constant1/1 -> compute_coeffs/3(mode)

== system libc_filters_diff/Var Discrete Filter (Zss c2d)/on_change ==
  in : Inport
  not equal : RelationalOperator  Operator=~=  OutDataTypeStr=boolean
  old : UnitDelay  InitialCondition=-1  SampleTime=-1
  has_changed : Outport
  wires:
  in/1 -> not equal/1, old/1
  old/1 -> not equal/2
  not equal/1 -> has_changed/1

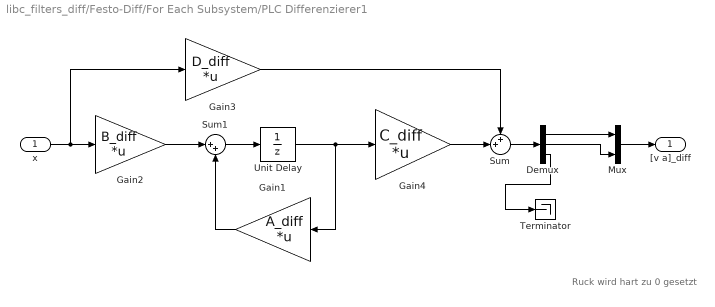
== system libc_filters_diff/Festo-Diff/For Each Subsystem/PLC Differenzierer1 ==
  note: Ruck wird hart zu 0 gesetzt
  x : Inport
  Demux : Demux  Outputs=3
  Gain1 : Gain  Gain=A_diff  Multiplication=Matrix(K*u)
  Gain2 : Gain  Gain=B_diff  Multiplication=Matrix(K*u)
  Gain3 : Gain  Gain=D_diff  Multiplication=Matrix(K*u)
  Gain4 : Gain  Gain=C_diff  Multiplication=Matrix(K*u)
  Mux : Mux  Inputs=2
  Sum : Sum  Inputs=++|
  Sum1 : Sum  Inputs=|++
  Terminator : Terminator
  Unit Delay : UnitDelay  InitialCondition=[0; 0; 0; 0]  SampleTime=-1
  "[v a]_diff" : Outport  PortDimensions=2
  wires:
  Gain1/1 -> Sum1/2
  Gain2/1 -> Sum1/1
  Gain3/1 -> Sum/1
  Gain4/1 -> Sum/2
  Sum1/1 -> Unit Delay/1
  Unit Delay/1 -> Gain4/1, Gain1/1
  x/1 -> Gain3/1, Gain2/1
  Sum/1 -> Demux/1
  Mux/1 -> "[v a]_diff"/1
  Demux/1 -> Mux/1
  Demux/2 -> Mux/2
  Demux/3 -> Terminator/1

== matlab function libc_filters_diff/2nd-Order Interpolation/2nd-Order Interpolation ==
  data: x0 input; x output; xE input; t input; T input
function x = smooth2nd(x0, xE, t, T)
%codegen
if T < 0
    T = 0;
end

if t < 0
    x = x0;
elseif t > T
    x = xE;
else
    if T == 0;
        x = xE;
    else
        dt = t/T;
        x = x0 + (xE - x0) .* (  10*dt^3 - 15*dt^4 + 6*dt^5  ); 
    end
end

== matlab function libc_filters_diff/Var Discrete Filter (Zss c2d)/compute_coeffs/compute_coeffs ==
  data: f input; tA input; cmode output; mode input; db output; cb output; ab output
function [cmode, db, cb, ab] = coeffs(f, tA, mode)
%#codegen

if tA == 0
    error('invalid sample time');
end
if f == 0
    error('invalid cut-off frequency');
end


cnum = 1;
cden = [1/(2*pi*f) 1];

dnum = [1, 1]; % default value
dden = [1, 1]; % default value
if mode == 3 % 'noh (d=0)'
    %[a,b,c,d]=tf2ss(cnum,cden); 
    %[ad,bd,cd,dd,~]=discret(-2*pi*f,2*pi*f,1,0,tA,'step_u',1e-9);
    a = -2*pi*f;
    b =  2*pi*f;
    c = 1;
    d = 0;
    t = tA;
    
    %[ad,bd] = c2d(a,b,tA);
    s = expm([[a b]*tA;zeros(1,2)]);
    ad = s(1,1);
    bd = s(1,2);
    
    
    
    dd = c*bd+d;
    bd = ad*bd;
    cd = c;
    mag_a = bode(a,b,c,d,1,62.8);
    mag_d = dbode(ad,bd,cd,dd,t,1,62.8);
    cd = cd*mag_a/mag_d;
    dd = dd*mag_a/mag_d;
        
    
    %[dnum,dden]=ss2tf(ad,bd,cd,dd,1);
    dnum = [dd, cd*bd - ad*dd];
    dden = [1, -ad];
    
end
if mode == 2 % 'foh (d=dt/2)'
    mode = 1;
    %d_sys = c2d(c_sys,tA,'foh');
    %[dnum,dden] = tfdata(d_sys,'v');
end
if mode == 1 % 'zoh (d=dt)'
    %d_sys = c2d(c_sys,tA);
    %[dnum,dden] = tfdata(d_sys,'v');
    %[dnum,dden] = c2d(-2*pi*f,2*pi*f,tA);
    a = -2*pi*f;
    b =  2*pi*f;
    t = tA;
    s = expm([[a b]*t;zeros(1,2)]);
    dnum = s(1,1);
    dden = s(1,2);
end

a = dden(2);
b = dden(1);
c = dnum(2);
d = dnum(1);

db = d/b;
cb = c/b;
ab = a/b;

cmode = mode;
